simulink model "TurtleBot3_GazeboDifferentialDriveControl"  (R2022b)
settings: Solver=VariableStepAuto  StartTime=0.0  StopTime=50  RelTol=1e-3
StopFcn:
  | robotPoses = out.yout{1}.Values.Data;
  | 
  | figure;
  | plot(waypoints(:,1), waypoints(:,2), 'k-x');
  | hold all
  | plot(robotPoses(:,1), robotPoses(:,2));
  | title('XY Waypoint Tracking');
undefined symbols (not defined in the file): duration, effort, Home1, Home2, index, joint_name, left_wheel_joint, model_name, right_wheel_joint, Target1, Target2, turtlebot3_burger, turtlebot3_burger_2
libraries: robotgazebolib x19, robotalgslib x2, robotcorelib x2
settings Model: PacingRate=0.011000  Creator=The MathWorks, Inc.  LastModifiedBy=Ismail
settings SolverCC: AlgebraicLoopSolver=TrustRegion
settings DebuggingCC: UnconnectedInputMsg=warning  UnconnectedOutputMsg=warning  UnconnectedLineMsg=warning  SymbolicDimsDataTypeCodeGenerationDiagnostic=none  SFMachineParentedDataDiag=warning
settings ModelReferenceCC: EnableRefExpFcnMdlSchedulingChecks=on

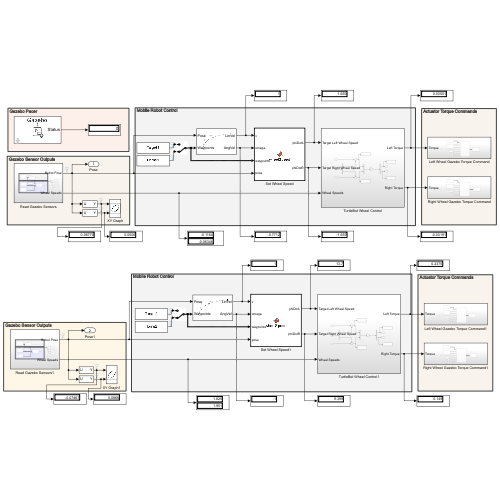
[thumbnail: Simulink's stored preview of the top-level diagram]
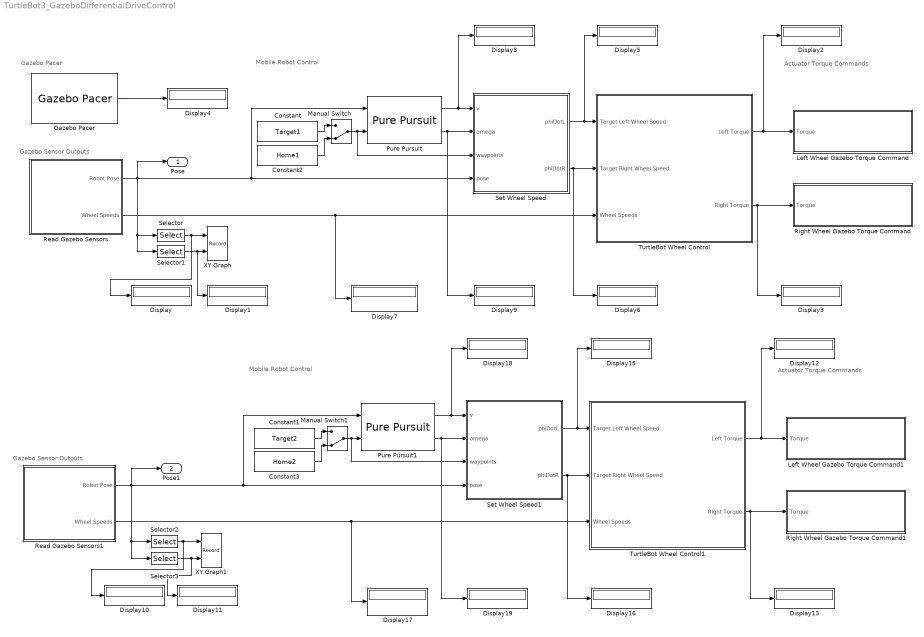
== system TurtleBot3_GazeboDifferentialDriveControl ==
  note: Gazebo Pacer
  note: Actuator Torque Commands
  note: Gazebo Sensor Outputs
  note: Mobile Robot Control
  note: Actuator Torque Commands
  note: Gazebo Sensor Outputs
  note: Mobile Robot Control
  Constant : Constant  Value=Target1
  Constant1 : Constant  Value=Target2
  Constant2 : Constant  Value=Home1
  Constant3 : Constant  Value=Home2
  Display{,1..13,15..19} (19 alike) : Display
  Gazebo Pacer : robotgazebolib/Gazebo Pacer  ResetBehavior=Reset Gazebo simulation time  SampleTime=0.01
  Left Wheel Gazebo Torque Command : Subsystem
  Left Wheel Gazebo Torque Command1 : Subsystem
  Manual Switch : ManualSwitch  CurrentSetting=0  varsize=on
  Manual Switch1 : ManualSwitch  CurrentSetting=0  varsize=on
  Pure Pursuit : robotalgslib/Pure Pursuit  DesiredLinearVelocity=1  MaxAngularVelocity=1  LookaheadDistance=0.2  TargetDirPort=off  SimulateUsing=Code generation
  Pure Pursuit1 : robotalgslib/Pure Pursuit  DesiredLinearVelocity=1  MaxAngularVelocity=1  LookaheadDistance=0.2  TargetDirPort=off  SimulateUsing=Code generation
  Read Gazebo Sensors : Subsystem
  Read Gazebo Sensors1 : Subsystem
  Right Wheel Gazebo Torque Command : Subsystem
  Right Wheel Gazebo Torque Command1 : Subsystem
  Selector : Selector  InputPortWidth=3  IndexOptions=Index vector (dialog)  Indices=[1]  OutputSizes=1
  Selector1 : Selector  InputPortWidth=3  IndexOptions=Index vector (dialog)  Indices=[2]  OutputSizes=1
  Selector2 : Selector  InputPortWidth=3  IndexOptions=Index vector (dialog)  Indices=[1]  OutputSizes=1
  Selector3 : Selector  InputPortWidth=3  IndexOptions=Index vector (dialog)  Indices=[2]  OutputSizes=1
  Set Wheel Speed : MATLAB Function  TreatAsAtomicUnit=on
  Set Wheel Speed1 : MATLAB Function  TreatAsAtomicUnit=on
  TurtleBot Wheel Control : Subsystem
  TurtleBot Wheel Control1 : Subsystem
  XY Graph : Record  FileSettingsInternal="{\"entries\":[{\"content\":{\"excelSettings\":{\"content\":{},\"type\":\"Streamout.ExcelSettings\"}},\"type\":\"Streamout.FileSettingStorage\",\"uuid\":\"9b76d6df-f2ee-41ae-a897-859777477549\"}],\"packageUris\":[\"http://schema.mathworks.com/mf0/streamout_blocks/R2020a\"],\"version\":\"1.0\"}"  Layout=[1 1]  SignalsInternal="{\"entries\":[{\"content\":{\"signals\":[{\"content\":{\"blockPath\":[\"TurtleBot3_GazeboDifferentialDriveControl/XY Graph\"],\"channel\":[],\"dimensions\":[1],\"domain\":\"TurtleBot3_GazeboDifferentialDriveControl/XY Graph\",\"lineColor\":\"#a2142f\",\"plots\":[1],\"port\":1,\"sid\":[\"\"],\"signalID\":45,\"signalName\":\"Selector\"},\"type\":\"RecordBlkView.Signal\",\"uuid\":\"7043024c-e0bb-448a-8998-882d1dee7e41\"},{\"content\":{\"blockPath\":[\"TurtleBot3_GazeboDifferentialDriveControl/XY Graph\"],\"channel\":[],\"dimensions\":[1],\"domain\":\"TurtleBot3_GazeboDifferentialDriveControl/XY Graph\",\"lineColor\":\"#a2142f\",\"plots\":[1],\"port\":2,\"sid\":[\"\"],\"signalID\":49,\"signalName\":\"Selector1\"},\"type\":\"RecordBlkView.Signal\",\"uuid\":\"b3c51245-1a48-4339-a3b7-0412a9798b1e\"}]},\"type\":\"RecordBlkView.InputSignals\",\"uuid\":\"7e430c38-4b51-4b74-b990-9fa0bdcf9de1\"}],\"packageUris\":[\"http://schema.mathworks.com/mf0/streamout_blocks/R2020a\"],\"version\":\"1.0\"}"  VisualizationBindings="{\"xyplotplugin\":{\"info\":[{\"series\":[{\"bindingParametersList\":[{\"parameter\":\"X-Axis\",\"signalID\":45,\"signalName\":\"Selector\"},{\"parameter\":\"Y-Axis\",\"signalID\":49,\"signalName\":\"Selector1\"}],\"seriesID\":8786}],\"subplotID\":1}]}}"  CompatibilityTag=XY  st=-1
  XY Graph1 : Record  FileSettingsInternal="{\"entries\":[{\"content\":{\"excelSettings\":{\"content\":{},\"type\":\"Streamout.ExcelSettings\"}},\"type\":\"Streamout.FileSettingStorage\",\"uuid\":\"365f15dd-1235-4737-b409-36fc80b55155\"}],\"packageUris\":[\"http://schema.mathworks.com/mf0/streamout_blocks/R2020a\"],\"version\":\"1.0\"}"  Layout=[1 1]  SignalsInternal="{\"entries\":[{\"content\":{\"signals\":[{\"content\":{\"blockPath\":[\"TurtleBot3_GazeboDifferentialDriveControl/XY Graph1\"],\"channel\":[],\"dimensions\":[1],\"domain\":\"TurtleBot3_GazeboDifferentialDriveControl/XY Graph1\",\"lineColor\":\"#0072bd\",\"plots\":[1],\"port\":1,\"sid\":[\"\"],\"signalID\":71,\"signalName\":\"Selector2\"},\"type\":\"RecordBlkView.Signal\",\"uuid\":\"75e92f67-50e1-4949-aba3-fae04aa0850f\"},{\"content\":{\"blockPath\":[\"TurtleBot3_GazeboDifferentialDriveControl/XY Graph1\"],\"channel\":[],\"dimensions\":[1],\"domain\":\"TurtleBot3_GazeboDifferentialDriveControl/XY Graph1\",\"lineColor\":\"#0072bd\",\"plots\":[1],\"port\":2,\"sid\":[\"\"],\"signalID\":75,\"signalName\":\"Selector3\"},\"type\":\"RecordBlkView.Signal\",\"uuid\":\"cd9207ee-1104-4a45-84ea-278db2908e9b\"}]},\"type\":\"RecordBlkView.InputSignals\",\"uuid\":\"dde98c37-01ab-40d2-bb84-96a6fb5361ec\"}],\"packageUris\":[\"http://schema.mathworks.com/mf0/streamout_blocks/R2020a\"],\"version\":\"1.0\"}"  VisualizationBindings="{\"xyplotplugin\":{\"info\":[{\"series\":[{\"bindingParametersList\":[{\"parameter\":\"X-Axis\",\"signalID\":71,\"signalName\":\"Selector2\"},{\"parameter\":\"Y-Axis\",\"signalID\":75,\"signalName\":\"Selector3\"}],\"seriesID\":2754}],\"subplotID\":1}]}}"  CompatibilityTag=XY  st=-1
  Pose : Outport
  Pose1 : Outport  Port=2
  wires:
  Set Wheel Speed/1(phiDotL) -> Display5/1, TurtleBot Wheel Control/1(Target Left Wheel Speed)
  Gazebo Pacer/1 -> Display4/1
  Read Gazebo Sensors/1(Robot Pose) -> Pose/1, Selector/1, Selector1/1, Pure Pursuit/1, Set Wheel Speed/4(pose)
  TurtleBot Wheel Control/1(Left Torque) -> Left Wheel Gazebo Torque Command/1(Torque), Display2/1
  TurtleBot Wheel Control/2(Right Torque) -> Display3/1, Right Wheel Gazebo Torque Command/1(Torque)
  Read Gazebo Sensors/2(Wheel Speeds) -> TurtleBot Wheel Control/3(Wheel Speeds), Display7/1
  Selector/1 -> XY Graph/1, Display/1
  Selector1/1 -> Display1/1, XY Graph/2
  Pure Pursuit/1 -> Display8/1, Set Wheel Speed/1(v)
  Pure Pursuit/2 -> Set Wheel Speed/2(omega), Display9/1
  Set Wheel Speed/2(phiDotR) -> Display6/1, TurtleBot Wheel Control/2(Target Right Wheel Speed)
  Read Gazebo Sensors1/1(Robot Pose) -> Pose1/1, Selector2/1, Selector3/1, Set Wheel Speed1/4(pose), Pure Pursuit1/1
  Selector3/1 -> Display11/1, XY Graph1/2
  Selector2/1 -> XY Graph1/1, Display10/1
  Read Gazebo Sensors1/2(Wheel Speeds) -> Display17/1, TurtleBot Wheel Control1/3(Wheel Speeds)
  Pure Pursuit1/1 -> Display18/1, Set Wheel Speed1/1(v)
  Pure Pursuit1/2 -> Set Wheel Speed1/2(omega), Display19/1
  TurtleBot Wheel Control1/2(Right Torque) -> Display13/1, Right Wheel Gazebo Torque Command1/1(Torque)
  TurtleBot Wheel Control1/1(Left Torque) -> Display12/1, Left Wheel Gazebo Torque Command1/1(Torque)
  Set Wheel Speed1/2(phiDotR) -> Display16/1, TurtleBot Wheel Control1/2(Target Right Wheel Speed)
  Set Wheel Speed1/1(phiDotL) -> Display15/1, TurtleBot Wheel Control1/1(Target Left Wheel Speed)
  Manual Switch/1 -> Set Wheel Speed/3(waypoints), Pure Pursuit/2
  Constant/1 -> Manual Switch/1
  Constant2/1 -> Manual Switch/2
  Manual Switch1/1 -> Set Wheel Speed1/3(waypoints), Pure Pursuit1/2
  Constant1/1 -> Manual Switch1/1
  Constant3/1 -> Manual Switch1/2

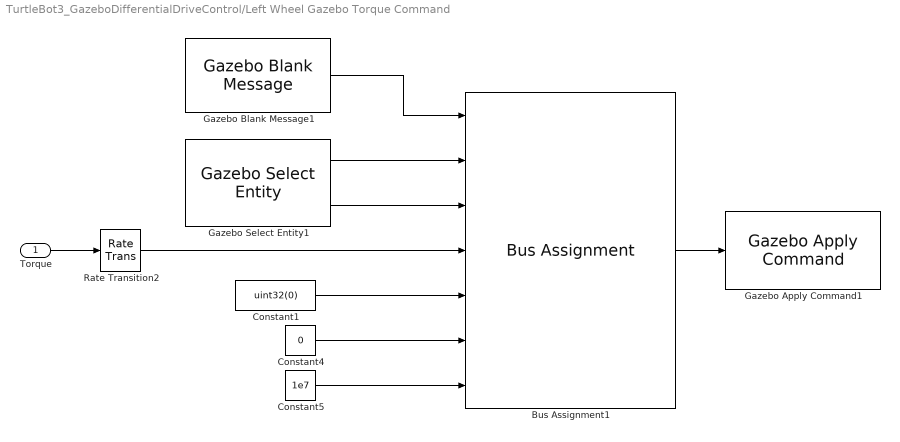
== system TurtleBot3_GazeboDifferentialDriveControl/Left Wheel Gazebo Torque Command ==
  Torque : Inport
  Bus Assignment1 : BusAssignment  AssignedSignals=model_name,joint_name,effort,index,duration.seconds,duration.nano_seconds
  Constant1 : Constant  Value=uint32(0)
  Constant4 : Constant  Value=0
  Constant5 : Constant  Value=1e7
  Gazebo Apply Command1 : robotgazebolib/Gazebo Apply Command  cmdType=ApplyJointTorque  sampleTime=0.01
  Gazebo Blank Message1 : robotgazebolib/Gazebo Blank Message  msgType=ApplyJointTorque  sampleTime=0.01  busName='Gazebo_SL_Bus_gazebo_msgs_ApplyJointTorque'
  Gazebo Select Entity1 : robotgazebolib/Gazebo Select Entity  modelElemName=turtlebot3_burger/left_wheel_joint  outputArraySize=128  OutputLabel=Joint  SelectType=Joint
  Rate Transition2 : RateTransition
  wires:
  Bus Assignment1/1 -> Gazebo Apply Command1/1
  Constant5/1 -> Bus Assignment1/7
  Gazebo Blank Message1/1 -> Bus Assignment1/1
  Gazebo Select Entity1/2 -> Bus Assignment1/3
  Gazebo Select Entity1/1 -> Bus Assignment1/2
  Torque/1 -> Rate Transition2/1
  Constant4/1 -> Bus Assignment1/6
  Rate Transition2/1 -> Bus Assignment1/4
  Constant1/1 -> Bus Assignment1/5

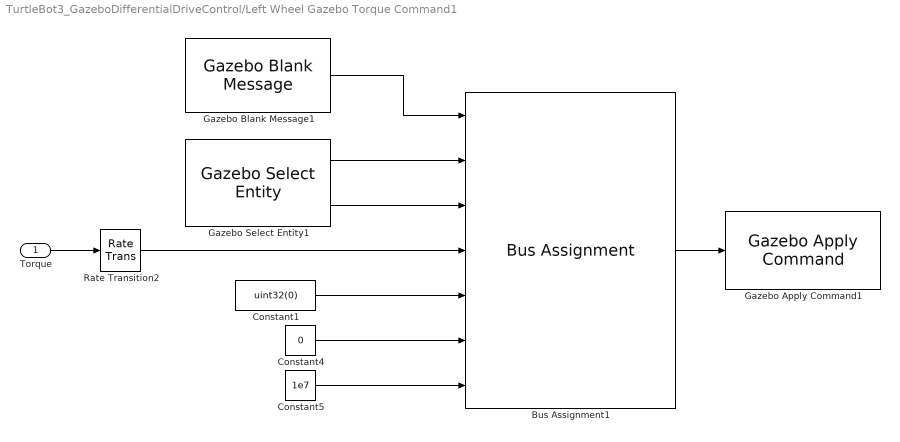
== system TurtleBot3_GazeboDifferentialDriveControl/Left Wheel Gazebo Torque Command1 ==
  Torque : Inport
  Bus Assignment1 : BusAssignment  AssignedSignals=model_name,joint_name,effort,index,duration.seconds,duration.nano_seconds
  Constant1 : Constant  Value=uint32(0)
  Constant4 : Constant  Value=0
  Constant5 : Constant  Value=1e7
  Gazebo Apply Command1 : robotgazebolib/Gazebo Apply Command  cmdType=ApplyJointTorque  sampleTime=0.01
  Gazebo Blank Message1 : robotgazebolib/Gazebo Blank Message  msgType=ApplyJointTorque  sampleTime=0.01  busName='Gazebo_SL_Bus_gazebo_msgs_ApplyJointTorque'
  Gazebo Select Entity1 : robotgazebolib/Gazebo Select Entity  modelElemName=turtlebot3_burger_2/left_wheel_joint  outputArraySize=128  OutputLabel=Joint  SelectType=Joint
  Rate Transition2 : RateTransition
  wires:
  Bus Assignment1/1 -> Gazebo Apply Command1/1
  Constant5/1 -> Bus Assignment1/7
  Gazebo Blank Message1/1 -> Bus Assignment1/1
  Gazebo Select Entity1/2 -> Bus Assignment1/3
  Gazebo Select Entity1/1 -> Bus Assignment1/2
  Torque/1 -> Rate Transition2/1
  Constant4/1 -> Bus Assignment1/6
  Rate Transition2/1 -> Bus Assignment1/4
  Constant1/1 -> Bus Assignment1/5

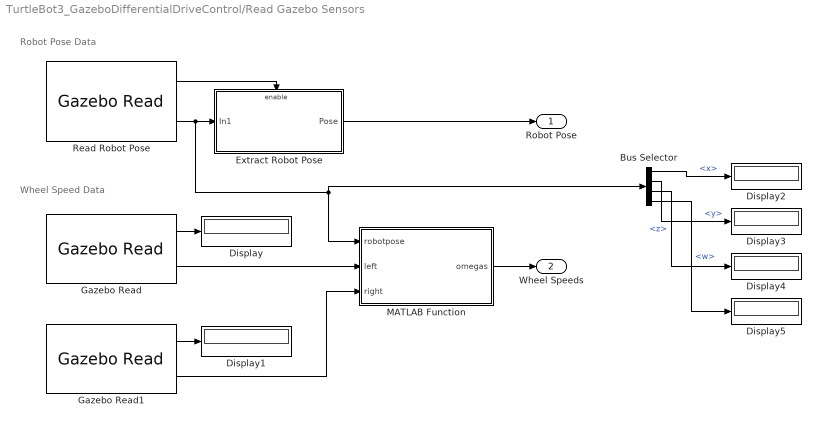
== system TurtleBot3_GazeboDifferentialDriveControl/Read Gazebo Sensors ==
  note: Robot Pose Data
  note: Wheel Speed Data
  Bus Selector : BusSelector  OutputSignals=orientation.x,orientation.y,orientation.z,orientation.w
  Display{,1..5} (6 alike) : Display
  Extract Robot Pose : Subsystem
  Gazebo Read : robotgazebolib/Gazebo Read  topicSource=From Gazebo  topic=/gazebo/ground_truth/world_pose/turtlebot3_burger/left_wheel  messageType=gazebo_msgs/Pose  sampleTime=0.01  fixedAxisBusStatus=off  jointAxisCount=2
  Gazebo Read1 : robotgazebolib/Gazebo Read  topicSource=From Gazebo  topic=/gazebo/ground_truth/world_pose/turtlebot3_burger/right_wheel  messageType=gazebo_msgs/Pose  sampleTime=0.01  fixedAxisBusStatus=off  jointAxisCount=2
  MATLAB Function : MATLAB Function  TreatAsAtomicUnit=on
  Read Robot Pose : robotgazebolib/Gazebo Read  topicSource=From Gazebo  topic=/gazebo/ground_truth/world_pose/turtlebot3_burger/base  messageType=gazebo_msgs/Pose  sampleTime=0.01  fixedAxisBusStatus=off  jointAxisCount=2
  Robot Pose : Outport
  Wheel Speeds : Outport  Port=2
  wires:
  Read Robot Pose/2 -> Bus Selector/1, MATLAB Function/1(robotpose), Extract Robot Pose/1(In1)
  Extract Robot Pose/1(Pose) -> Robot Pose/1
  Read Robot Pose/1 -> Extract Robot Pose/Enable
  Gazebo Read/1 -> Display/1
  Gazebo Read1/1 -> Display1/1
  MATLAB Function/1(omegas) -> Wheel Speeds/1
  Gazebo Read/2 -> MATLAB Function/2(left)
  Gazebo Read1/2 -> MATLAB Function/3(right)
  Bus Selector/1 -> Display2/1  "<x>"
  Bus Selector/4 -> Display5/1  "<w>"
  Bus Selector/3 -> Display4/1  "<z>"
  Bus Selector/2 -> Display3/1  "<y>"

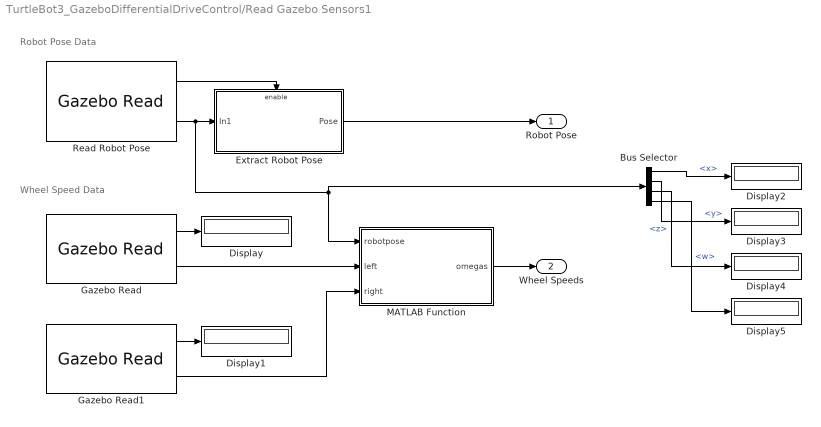
== system TurtleBot3_GazeboDifferentialDriveControl/Read Gazebo Sensors1 ==
  note: Robot Pose Data
  note: Wheel Speed Data
  Bus Selector : BusSelector  OutputSignals=orientation.x,orientation.y,orientation.z,orientation.w
  Display{,1..5} (6 alike) : Display
  Extract Robot Pose : Subsystem
  Gazebo Read : robotgazebolib/Gazebo Read  topicSource=From Gazebo  topic=/gazebo/ground_truth/world_pose/turtlebot3_burger_2/left_wheel  messageType=gazebo_msgs/Pose  sampleTime=0.01  fixedAxisBusStatus=off  jointAxisCount=2
  Gazebo Read1 : robotgazebolib/Gazebo Read  topicSource=From Gazebo  topic=/gazebo/ground_truth/world_pose/turtlebot3_burger_2/right_wheel  messageType=gazebo_msgs/Pose  sampleTime=0.01  fixedAxisBusStatus=off  jointAxisCount=2
  MATLAB Function : MATLAB Function  TreatAsAtomicUnit=on
  Read Robot Pose : robotgazebolib/Gazebo Read  topicSource=From Gazebo  topic=/gazebo/ground_truth/world_pose/turtlebot3_burger_2/base  messageType=gazebo_msgs/Pose  sampleTime=0.01  fixedAxisBusStatus=off  jointAxisCount=2
  Robot Pose : Outport
  Wheel Speeds : Outport  Port=2
  wires:
  Read Robot Pose/2 -> Bus Selector/1, MATLAB Function/1(robotpose), Extract Robot Pose/1(In1)
  Extract Robot Pose/1(Pose) -> Robot Pose/1
  Read Robot Pose/1 -> Extract Robot Pose/Enable
  Gazebo Read/1 -> Display/1
  Gazebo Read1/1 -> Display1/1
  MATLAB Function/1(omegas) -> Wheel Speeds/1
  Gazebo Read/2 -> MATLAB Function/2(left)
  Gazebo Read1/2 -> MATLAB Function/3(right)
  Bus Selector/1 -> Display2/1  "<x>"
  Bus Selector/4 -> Display5/1  "<w>"
  Bus Selector/3 -> Display4/1  "<z>"
  Bus Selector/2 -> Display3/1  "<y>"

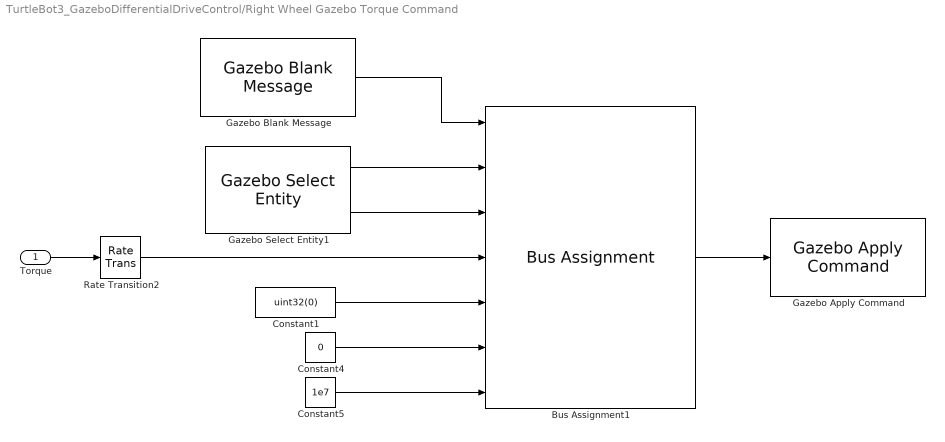
== system TurtleBot3_GazeboDifferentialDriveControl/Right Wheel Gazebo Torque Command ==
  Torque : Inport
  Bus Assignment1 : BusAssignment  AssignedSignals=model_name,joint_name,effort,index,duration.seconds,duration.nano_seconds
  Constant1 : Constant  Value=uint32(0)
  Constant4 : Constant  Value=0
  Constant5 : Constant  Value=1e7
  Gazebo Apply Command : robotgazebolib/Gazebo Apply Command  cmdType=ApplyJointTorque  sampleTime=0.01
  Gazebo Blank Message : robotgazebolib/Gazebo Blank Message  msgType=ApplyJointTorque  sampleTime=0.01  busName='Gazebo_SL_Bus_gazebo_msgs_ApplyJointTorque'
  Gazebo Select Entity1 : robotgazebolib/Gazebo Select Entity  modelElemName=turtlebot3_burger/right_wheel_joint  outputArraySize=128  OutputLabel=Joint  SelectType=Joint
  Rate Transition2 : RateTransition
  wires:
  Constant1/1 -> Bus Assignment1/5
  Rate Transition2/1 -> Bus Assignment1/4
  Constant4/1 -> Bus Assignment1/6
  Torque/1 -> Rate Transition2/1
  Gazebo Select Entity1/1 -> Bus Assignment1/2
  Gazebo Select Entity1/2 -> Bus Assignment1/3
  Gazebo Blank Message/1 -> Bus Assignment1/1
  Constant5/1 -> Bus Assignment1/7
  Bus Assignment1/1 -> Gazebo Apply Command/1

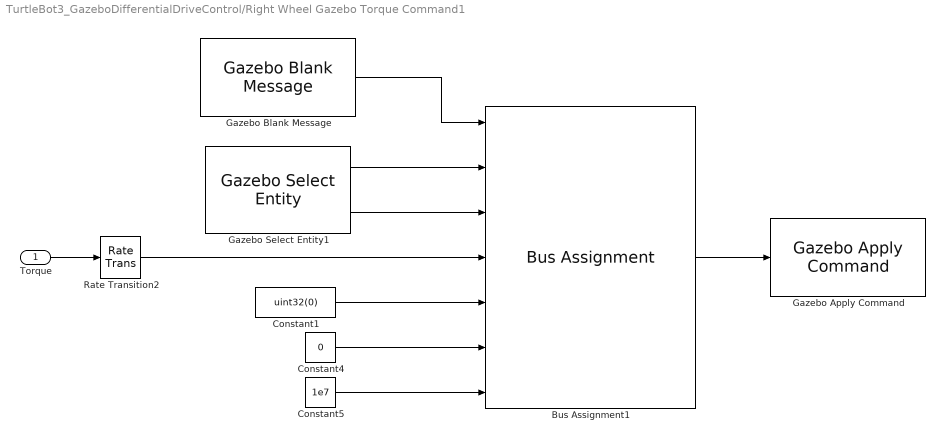
== system TurtleBot3_GazeboDifferentialDriveControl/Right Wheel Gazebo Torque Command1 ==
  Torque : Inport
  Bus Assignment1 : BusAssignment  AssignedSignals=model_name,joint_name,effort,index,duration.seconds,duration.nano_seconds
  Constant1 : Constant  Value=uint32(0)
  Constant4 : Constant  Value=0
  Constant5 : Constant  Value=1e7
  Gazebo Apply Command : robotgazebolib/Gazebo Apply Command  cmdType=ApplyJointTorque  sampleTime=0.01
  Gazebo Blank Message : robotgazebolib/Gazebo Blank Message  msgType=ApplyJointTorque  sampleTime=0.01  busName='Gazebo_SL_Bus_gazebo_msgs_ApplyJointTorque'
  Gazebo Select Entity1 : robotgazebolib/Gazebo Select Entity  modelElemName=turtlebot3_burger_2/right_wheel_joint  outputArraySize=128  OutputLabel=Joint  SelectType=Joint
  Rate Transition2 : RateTransition
  wires:
  Constant1/1 -> Bus Assignment1/5
  Rate Transition2/1 -> Bus Assignment1/4
  Constant4/1 -> Bus Assignment1/6
  Torque/1 -> Rate Transition2/1
  Gazebo Select Entity1/1 -> Bus Assignment1/2
  Gazebo Select Entity1/2 -> Bus Assignment1/3
  Gazebo Blank Message/1 -> Bus Assignment1/1
  Constant5/1 -> Bus Assignment1/7
  Bus Assignment1/1 -> Gazebo Apply Command/1

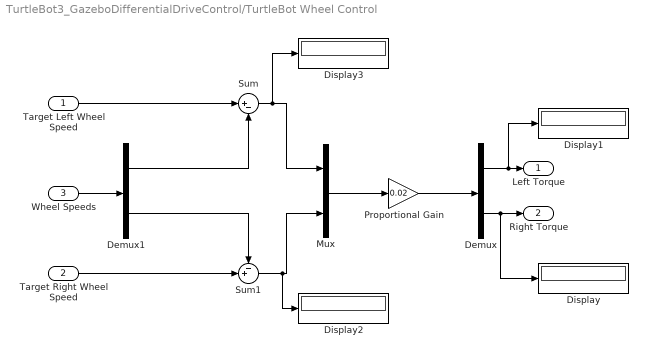
== system TurtleBot3_GazeboDifferentialDriveControl/TurtleBot Wheel Control ==
  Target Left Wheel Speed : Inport
  Target Right Wheel Speed : Inport  Port=2
  Wheel Speeds : Inport  Port=3
  Demux : Demux  Outputs=2
  Demux1 : Demux  Outputs=2
  Display{,1..3} (4 alike) : Display
  Mux : Mux  Inputs=2
  Proportional Gain : Gain  Gain=0.02
  Sum : Sum  Inputs=|+-
  Sum1 : Sum  Inputs=-+|
  Left Torque : Outport
  Right Torque : Outport  Port=2
  wires:
  Sum1/1 -> Display2/1, Mux/2
  Target Left Wheel Speed/1 -> Sum/1
  Sum/1 -> Display3/1, Mux/1
  Mux/1 -> Proportional Gain/1
  Proportional Gain/1 -> Demux/1
  Demux/1 -> Display1/1, Left Torque/1
  Wheel Speeds/1 -> Demux1/1
  Demux1/1 -> Sum/2
  Target Right Wheel Speed/1 -> Sum1/2
  Demux1/2 -> Sum1/1
  Demux/2 -> Display/1, Right Torque/1

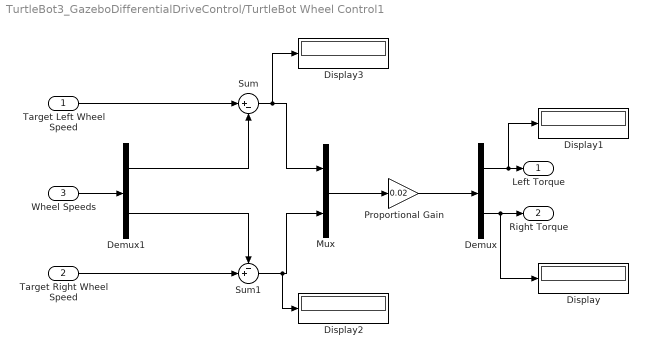
== system TurtleBot3_GazeboDifferentialDriveControl/TurtleBot Wheel Control1 ==
  Target Left Wheel Speed : Inport
  Target Right Wheel Speed : Inport  Port=2
  Wheel Speeds : Inport  Port=3
  Demux : Demux  Outputs=2
  Demux1 : Demux  Outputs=2
  Display{,1..3} (4 alike) : Display
  Mux : Mux  Inputs=2
  Proportional Gain : Gain  Gain=0.02
  Sum : Sum  Inputs=|+-
  Sum1 : Sum  Inputs=-+|
  Left Torque : Outport
  Right Torque : Outport  Port=2
  wires:
  Sum1/1 -> Display2/1, Mux/2
  Target Left Wheel Speed/1 -> Sum/1
  Sum/1 -> Display3/1, Mux/1
  Mux/1 -> Proportional Gain/1
  Proportional Gain/1 -> Demux/1
  Demux/1 -> Display1/1, Left Torque/1
  Wheel Speeds/1 -> Demux1/1
  Demux1/1 -> Sum/2
  Target Right Wheel Speed/1 -> Sum1/2
  Demux1/2 -> Sum1/1
  Demux/2 -> Display/1, Right Torque/1

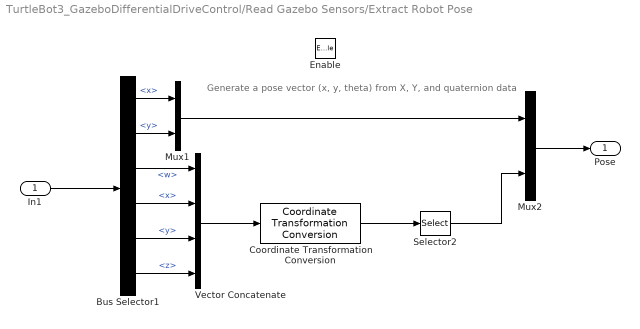
== system TurtleBot3_GazeboDifferentialDriveControl/Read Gazebo Sensors/Extract Robot Pose ==
  note: Generate a pose vector (x, y, theta) from X, Y, and quaternion data
  In1 : Inport
  Enable : EnablePort
  Bus Selector1 : BusSelector  OutputSignals=position.x,position.y,orientation.w,orientation.x,orientation.y,orientation.z
  Coordinate Transformation Conversion : robotcorelib/Coordinate Transformation Conversion  InputRepresentation=Quaternion  InputEulerSequence=ZYX  ShowTrVecInputPort=on  OutputRepresentation=Euler Angles  OutputEulerSequence=ZYX  ShowTrVecOutputPort=on  SimulateUsing=Interpreted execution
  Mux1 : Mux  Inputs=2
  Mux2 : Mux  Inputs=2
  Selector2 : Selector  InputPortWidth=3  IndexOptions=Index vector (dialog)  Indices=1  OutputSizes=1
  Vector Concatenate : Concatenate  NumInputs=4
  Pose : Outport  VectorParamsAs1DForOutWhenUnconnected=off
  wires:
  Vector Concatenate/1 -> Coordinate Transformation Conversion/1
  Coordinate Transformation Conversion/1 -> Selector2/1
  Mux1/1 -> Mux2/1
  Selector2/1 -> Mux2/2
  Mux2/1 -> Pose/1
  Bus Selector1/6 -> Vector Concatenate/4  "<z>"
  Bus Selector1/1 -> Mux1/1  "<x>"
  Bus Selector1/4 -> Vector Concatenate/2  "<x>"
  Bus Selector1/2 -> Mux1/2  "<y>"
  Bus Selector1/3 -> Vector Concatenate/1  "<w>"
  Bus Selector1/5 -> Vector Concatenate/3  "<y>"
  In1/1 -> Bus Selector1/1

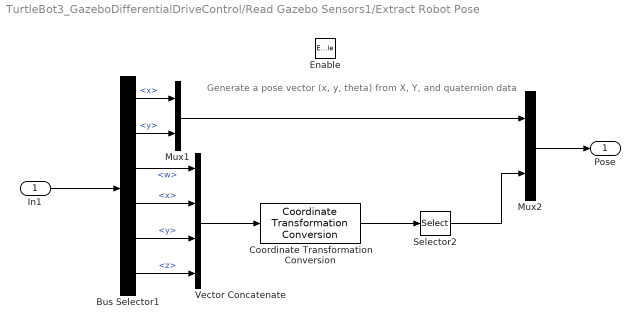
== system TurtleBot3_GazeboDifferentialDriveControl/Read Gazebo Sensors1/Extract Robot Pose ==
  note: Generate a pose vector (x, y, theta) from X, Y, and quaternion data
  In1 : Inport
  Enable : EnablePort
  Bus Selector1 : BusSelector  OutputSignals=position.x,position.y,orientation.w,orientation.x,orientation.y,orientation.z
  Coordinate Transformation Conversion : robotcorelib/Coordinate Transformation Conversion  InputRepresentation=Quaternion  InputEulerSequence=ZYX  ShowTrVecInputPort=on  OutputRepresentation=Euler Angles  OutputEulerSequence=ZYX  ShowTrVecOutputPort=on  SimulateUsing=Interpreted execution
  Mux1 : Mux  Inputs=2
  Mux2 : Mux  Inputs=2
  Selector2 : Selector  InputPortWidth=3  IndexOptions=Index vector (dialog)  Indices=1  OutputSizes=1
  Vector Concatenate : Concatenate  NumInputs=4
  Pose : Outport  VectorParamsAs1DForOutWhenUnconnected=off
  wires:
  Vector Concatenate/1 -> Coordinate Transformation Conversion/1
  Coordinate Transformation Conversion/1 -> Selector2/1
  Mux1/1 -> Mux2/1
  Selector2/1 -> Mux2/2
  Mux2/1 -> Pose/1
  Bus Selector1/6 -> Vector Concatenate/4  "<z>"
  Bus Selector1/1 -> Mux1/1  "<x>"
  Bus Selector1/4 -> Vector Concatenate/2  "<x>"
  Bus Selector1/2 -> Mux1/2  "<y>"
  Bus Selector1/3 -> Vector Concatenate/1  "<w>"
  Bus Selector1/5 -> Vector Concatenate/3  "<y>"
  In1/1 -> Bus Selector1/1

== matlab function TurtleBot3_GazeboDifferentialDriveControl/Read Gazebo Sensors/MATLAB Function ==
  data: robotpose input; omegas output; left input; right input
function omegas = computeWheelVelocities(robotpose, left, right)
%computeWheelVelocities computes wheel velocity based on rate of change of
%the yaw angle of the wheel relative to its original mount on the robot
%body

persistent initAngles
if isempty(initAngles)
    initAngles = zeros(2,1);
end
sampleTime = 0.01;

% compute rotation between wheel original mount on the robot body and world
% frame
robotRtom = quat2rotm([robotpose.orientation.w, robotpose.orientation.x, robotpose.orientation.y, robotpose.orientation.z]);
originalWheelMount = robotRtom*eul2rotm([pi/2 pi/2 0]);

% get rotation between wheel and the world frame
leftRtom = quat2rotm([left.orientation.w, left.orientation.x, left.orientation.y, left.orientation.z]);
rightRtom = quat2rotm([right.orientation.w, right.orientation.x, right.orientation.y, right.orientation.z]);

% compute relative rotation between wheel and its original mount
leftRotation = rotm2eul(originalWheelMount'*leftRtom);
rightRotation = rotm2eul(originalWheelMount'*rightRtom);

% compute angluar velocity using the angle difference between the current
% angle pose and the the angle pose in last time step
angles = [leftRotation(1); rightRotation(1)];
omegas = angdiff(initAngles, angles)/sampleTime;
initAngles = angles;

== matlab function TurtleBot3_GazeboDifferentialDriveControl/Set Wheel Speed ==
  data: v input; omega input; waypoints input; pose input; phiDotL output; phiDotR output
function [phiDotL, phiDotR] = wheelSpeed(v, omega, waypoints, pose)

% Path constants
stopThreshold = 0.1;
slowThreshold = 0.3;

% Robot constants
trackWidth = 0.142;%0.381;
wheelRadius = 0.033;%0.195/2;

% Slow the robot down when it's near the threshold
distanceToEndpoint = norm(waypoints(end, :) - pose(1:2)');
if (distanceToEndpoint < slowThreshold)
    v = distanceToEndpoint/slowThreshold*v;
    
    % Stop the robot if it's inside the target threshold
    if distanceToEndpoint < stopThreshold
        v = 0;
    end
end

% Convert velocity and heading angular velocity to wheel speeds
phiDotL = (v - trackWidth/2*omega)/wheelRadius;
phiDotR = (v + trackWidth/2*omega)/wheelRadius;

end

== matlab function TurtleBot3_GazeboDifferentialDriveControl/Read Gazebo Sensors1/MATLAB Function ==
  data: robotpose input; omegas output; left input; right input
function omegas = computeWheelVelocities(robotpose, left, right)
%computeWheelVelocities computes wheel velocity based on rate of change of
%the yaw angle of the wheel relative to its original mount on the robot
%body

persistent initAngles
if isempty(initAngles)
    initAngles = zeros(2,1);
end
sampleTime = 0.01;

% compute rotation between wheel original mount on the robot body and world
% frame
robotRtom = quat2rotm([robotpose.orientation.w, robotpose.orientation.x, robotpose.orientation.y, robotpose.orientation.z]);
originalWheelMount = robotRtom*eul2rotm([pi/2 pi/2 0]);

% get rotation between wheel and the world frame
leftRtom = quat2rotm([left.orientation.w, left.orientation.x, left.orientation.y, left.orientation.z]);
rightRtom = quat2rotm([right.orientation.w, right.orientation.x, right.orientation.y, right.orientation.z]);

% compute relative rotation between wheel and its original mount
leftRotation = rotm2eul(originalWheelMount'*leftRtom);
rightRotation = rotm2eul(originalWheelMount'*rightRtom);

% compute angluar velocity using the angle difference between the current
% angle pose and the the angle pose in last time step
angles = [leftRotation(1); rightRotation(1)];
omegas = angdiff(initAngles, angles)/sampleTime;
initAngles = angles;

== matlab function TurtleBot3_GazeboDifferentialDriveControl/Set Wheel Speed1 ==
  data: v input; omega input; waypoints input; pose input; phiDotL output; phiDotR output
function [phiDotL, phiDotR] = wheelSpeed(v, omega, waypoints, pose)

% Path constants
stopThreshold = 0.1;
slowThreshold = 0.3;

% Robot constants
trackWidth = 0.142;%0.381;
wheelRadius = 0.033;%0.195/2;

% Slow the robot down when it's near the threshold
distanceToEndpoint = norm(waypoints(end, :) - pose(1:2)');
if (distanceToEndpoint < slowThreshold)
    v = distanceToEndpoint/slowThreshold*v;
    
    % Stop the robot if it's inside the target threshold
    if distanceToEndpoint < stopThreshold
        v = 0;
    end
end

% Convert velocity and heading angular velocity to wheel speeds
phiDotL = (v - trackWidth/2*omega)/wheelRadius;
phiDotR = (v + trackWidth/2*omega)/wheelRadius;

end
